simulink model "Project_4_Simulation"  (R2023b)
settings: Solver=VariableStepAuto  StartTime=0.0  StopTime=10.0  RelTol=1e-3
undefined symbols (not defined in the file or in its folder): batData, carData, motorData, track_radius
libraries: slpidlib x1
settings Model: Creator=mccal  LastModifiedBy=mccal

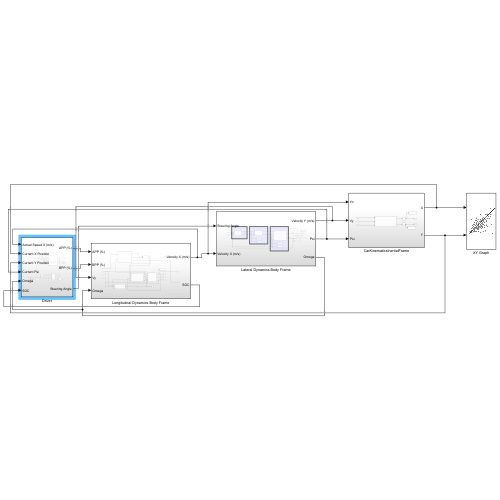
[thumbnail: Simulink's stored preview of the top-level diagram]
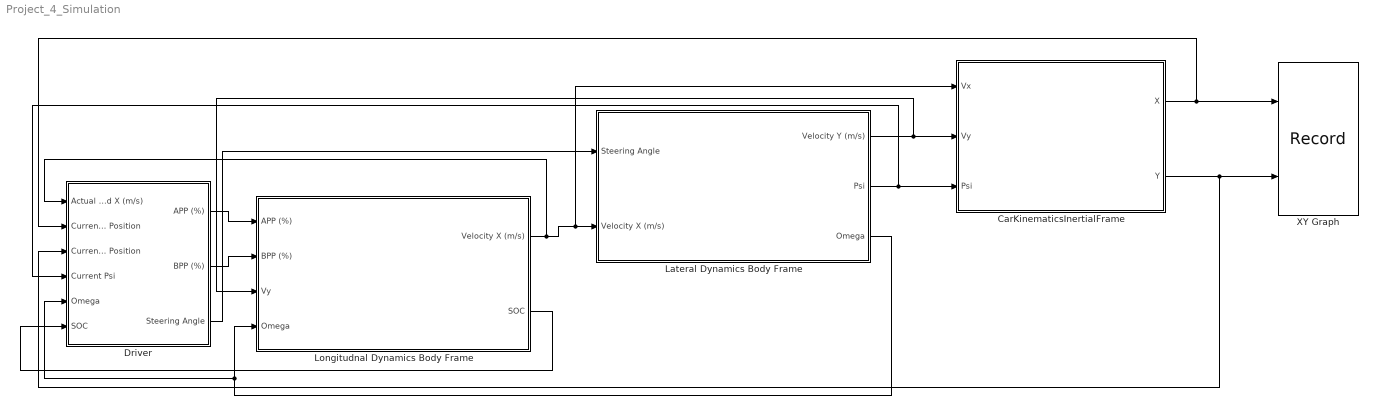
== system Project_4_Simulation ==
  CarKinematicsInertialFrame : Subsystem
  Driver : Subsystem
  Lateral Dynamics Body Frame : Subsystem
  Longitudnal Dynamics Body Frame : Subsystem
  XY Graph : Record  FileSettingsInternal="{\"entries\":[{\"content\":{\"excelSettings\":{\"content\":{},\"type\":\"Streamout.ExcelSettings\"}},\"type\":\"Streamout.FileSettingStorage\",\"uuid\":\"\"}],\"packageUris\":[\"http:\\/\\/schema.mathworks.com\\/mf0\\/streamout_blocks\\/R2020a\"],\"version\":\"1.0\"}"  Layout=[1 1]  SignalsInternal="{\"entries\":[{\"content\":{\"signals\":[{\"content\":{\"blockPath\":[],\"dimensions\":[1],\"domain\":\"\",\"lineColor\":\"#d95319\",\"port\":1,\"sid\":[\"\"],\"signalID\":3841,\"signalName\":\"CarKinematicsInertialFrame:1\"},\"type\":\"RecordBlkView.Signal\",\"uuid\":\"\"},{\"content\":{\"blockPath\":[],\"dimensions\":[1],\"domain\":\"\",\"lineColor\":\"#edb120\",\"port\":2,\"sid\":[\"\"],\"signalID\":3845,\"signalName\":\"CarKinematicsInertialFrame:2\"},\"type\":\"RecordBlkView.Signal\",\"uuid\":\"\"}]},\"type\":\"RecordBlkView.InputSignals\",\"uuid\":\"\"}],\"packageUris\":[\"http:\\/\\/schema.mathworks.com\\/mf0\\/streamout_blocks\\/R2020a\"],\"version\":\"1.0\"}"  VisualizationBindings="{\"xyplotplugin\":{\"info\":[{\"series\":[],\"subplotID\":1}]}}"  CompatibilityTag=XY  st=-1
  wires:
  CarKinematicsInertialFrame/2(Y) -> Driver/3(Current Y Position), XY Graph/2
  CarKinematicsInertialFrame/1(X) -> Driver/2(Current X Position), XY Graph/1
  Lateral Dynamics Body Frame/1(Velocity Y (m/s)) -> Longitudnal Dynamics Body Frame/3(Vy), CarKinematicsInertialFrame/2(Vy)
  Lateral Dynamics Body Frame/2(Psi) -> Driver/4(Current Psi), CarKinematicsInertialFrame/3(Psi)
  Driver/1(APP (%)) -> Longitudnal Dynamics Body Frame/1(APP (%))
  Driver/2(BPP (%)) -> Longitudnal Dynamics Body Frame/2(BPP (%))
  Longitudnal Dynamics Body Frame/1(Velocity X (m/s)) -> Driver/1(Actual Speed X (m/s)), CarKinematicsInertialFrame/1(Vx), Lateral Dynamics Body Frame/2(Velocity X (m/s))
  Lateral Dynamics Body Frame/3(Omega) -> Longitudnal Dynamics Body Frame/4(Omega), Driver/5(Omega)
  Longitudnal Dynamics Body Frame/2(SOC) -> Driver/6(SOC)
  Driver/3(Steering Angle) -> Lateral Dynamics Body Frame/1(Steering Angle)

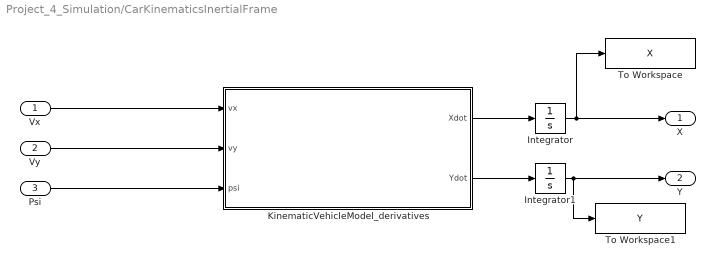
== system Project_4_Simulation/CarKinematicsInertialFrame ==
  Vx : Inport
  Vy : Inport  Port=2
  Psi : Inport  Port=3
  Integrator : Integrator  InitialCondition=carData.init.X0
  Integrator1 : Integrator  InitialCondition=carData.init.Y0
  KinematicVehicleModel_derivatives : MATLAB Function  TreatAsAtomicUnit=on  mask{obj=carData}
      mask prompts: obj "obj structure"
  To Workspace : ToWorkspace  VariableName=X  SaveFormat=Timeseries  SampleTime=-1
  To Workspace1 : ToWorkspace  VariableName=Y  SaveFormat=Timeseries  SampleTime=-1
  X : Outport
  Y : Outport  Port=2
  wires:
  KinematicVehicleModel_derivatives/1(Xdot) -> Integrator/1
  KinematicVehicleModel_derivatives/2(Ydot) -> Integrator1/1
  Integrator/1 -> To Workspace/1, X/1
  Integrator1/1 -> To Workspace1/1, Y/1
  Vx/1 -> KinematicVehicleModel_derivatives/1(vx)
  Vy/1 -> KinematicVehicleModel_derivatives/2(vy)
  Psi/1 -> KinematicVehicleModel_derivatives/3(psi)

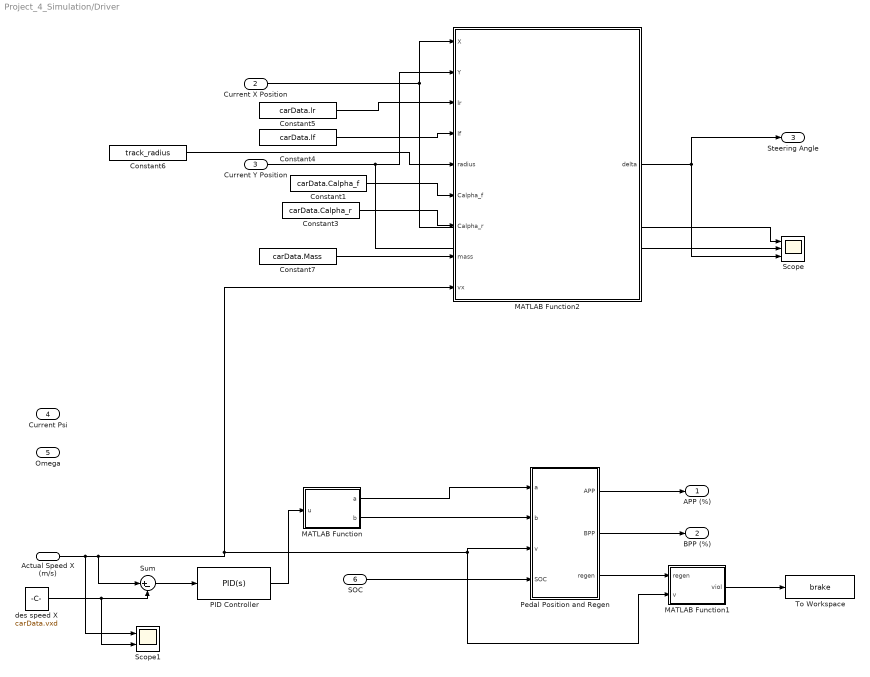
== system Project_4_Simulation/Driver ==
  Actual Speed X (m/s) : Inport
  Current X Position : Inport  Port=2
  Current Y Position : Inport  Port=3
  Current Psi : Inport  Port=4
  Omega : Inport  Port=5
  SOC : Inport  Port=6
  Constant1 : Constant  Value=carData.Calpha_f
  Constant3 : Constant  Value=carData.Calpha_r
  Constant4 : Constant  Value=carData.lf
  Constant5 : Constant  Value=carData.lr
  Constant6 : Constant  Value=track_radius
  Constant7 : Constant  Value=carData.Mass
  MATLAB Function : MATLAB Function  TreatAsAtomicUnit=on
  MATLAB Function1 : MATLAB Function  TreatAsAtomicUnit=on
  MATLAB Function2 : MATLAB Function  TreatAsAtomicUnit=on
  PID Controller : slpidlib/PID Controller  Controller=PID  Form=Parallel  TimeDomain=Continuous-time  UseExternalTs=off  SampleTime=-1  IntegratorMethod=Forward Euler  FilterMethod=Forward Euler  ControllerParametersSource=internal  P=1  I=0  UseKiTs=off  D=0  N=100  UseFilter=on  TunerSelectOption=Transfer Function Based (PID Tuner App)  InitialConditionSource=internal  InitialConditionForIntegrator=0  InitialConditionForFilter=0  DifferentiatorICPrevScaledInput=0  ExternalReset=none  TrackingMode=off  Kt=1  LimitOutput=on  SatLimitsSource=internal  UpperSaturationLimit=1  LowerSaturationLimit=-1  LinearizeAsGain=off  AntiWindupMode=none  Kb=1  LimitIntegrator=off  UpperIntegratorSaturationLimit=inf  LowerIntegratorSaturationLimit=-inf  POutMin=[]  POutMax=[]  IOutMin=[]  IOutMax=[]  DOutMin=[]  DOutMax=[]  NOutMin=[]  NOutMax=[]  SumOutMin=[]  SumOutMax=[]  SaturationOutMin=[]  SaturationOutMax=[]  PParamMin=[]  PParamMax=[]  IParamMin=[]  IParamMax=[]  DParamMin=[]  DParamMax=[]  NParamMin=[]  NParamMax=[]  KbParamMin=[]  KbParamMax=[]  KtParamMin=[]  KtParamMax=[]  KbOutMin=[]  KbOutMax=[]  KtOutMin=[]  KtOutMax=[]  IntegratorOutMin=[]  IntegratorOutMax=[]  FilterOutMin=[]  FilterOutMax=[]  SumI1OutMin=[]  SumI1OutMax=[]  SumI2OutMin=[]  SumI2OutMax=[]  SumI3OutMin=[]  SumI3OutMax=[]  SumI4OutMin=[]  SumI4OutMax=[]  SumDOutMin=[]  SumDOutMax=[]  DifferentiatorOutMin=[]  DifferentiatorOutMax=[]  FilterDiffOutCoefMin=[]  FilterDiffOutCoefMax=[]  ReciprocalOutMin=[]  ReciprocalOutMax=[]  SumDenOutMin=[]  SumDenOutMax=[]  SumNumOutMin=[]  SumNumOutMax=[]  DivideOutMin=[]  DivideOutMax=[]  UdiffTsProdOutMin=[]  UdiffTsProdOutMax=[]  NTsProdOutMin=[]  NTsProdOutMax=[]  UintegralTsProdOutMin=[]  UintegralTsProdOutMax=[]  UngainTsProdOutMin=[]  UngainTsProdOutMax=[]  ClampingZeroOutDataTypeStr=Inherit: Inherit via back propagation  ClampingZeroOutMin=[]  ClampingZeroOutMax=[]  FilterDenConstantOutDataTypeStr=Inherit: Inherit via back propagation  FilterDenConstantOutMin=[]  FilterDenConstantOutMax=[]  PCopyOutDataTypeStr=Inherit: Inherit via back propagation  PCopyOutMin=[]  PCopyOutMax=[]  NCopyOutDataTypeStr=Inherit: Inherit via back propagation  NCopyOutMin=[]  NCopyOutMax=[]  IntegratorContinuousStateAttributes=''  IntegratorStateMustResolveToSignalObject=off  IntegratorRTWStateStorageClass=Auto  FilterContinuousStateAttributes=''  FilterStateMustResolveToSignalObject=off  FilterRTWStateStorageClass=Auto  ParallelPVariant=InternalParameters  IdealPVariant=Disabled  IVariant=InternalParameters  DVariant=InternalParameters  IntegratorVariant=Continuous  SatVariant=Enabled  AWVariant=Passthrough  PCopyVariant=Disabled  TRVariant=Disabled  FdbkBlocksVariant=Forward  IdealPFdbkVariant=Disabled  SatFdbkVariant=Disabled  DerivativeFilterVariant=ContFilter  NVariant=InternalParameters  NCopyVariant=Disabled  FilterICVariant=InternalICsFilter  IntegratorICVariant=InternalICs  ExternalResetVariant=Disabled  TRSumVariant=Passthrough  SumFdbkVariant=Disabled  SumVariant=Sum_PID  TsampFilterVariant=InternalTs  TsampNgainVariant=Passthrough  TsampIntegralVariant=Disabled_SignalSpec  ExternalSaturationOutDataTypeStr=Inherit: Same as second input
  Pedal Position and Regen : MATLAB Function  TreatAsAtomicUnit=on
  Scope : Scope  NumInputPorts=3
  Scope1 : Scope  NumInputPorts=2
  Sum : Sum  Inputs=|+-
  To Workspace : ToWorkspace  VariableName=brake  SaveFormat=Timeseries  SampleTime=-1
  des speed X : Constant  Value=carData.vxd
  APP (%) : Outport
  BPP (%) : Outport  Port=2
  Steering Angle : Outport  Port=3
  wires:
  Pedal Position and Regen/1(APP) -> APP (%)/1
  Pedal Position and Regen/2(BPP) -> BPP (%)/1
  Pedal Position and Regen/3(regen) -> MATLAB Function1/1(regen)
  MATLAB Function1/1(viol) -> To Workspace/1
  Current X Position/1 -> Scope/1, MATLAB Function2/1(X)
  Constant3/1 -> MATLAB Function2/7(Calpha_r)
  Current Y Position/1 -> Scope/2, MATLAB Function2/2(Y)
  Constant1/1 -> MATLAB Function2/6(Calpha_f)
  Constant6/1 -> MATLAB Function2/5(radius)
  Constant5/1 -> MATLAB Function2/3(lr)
  Constant7/1 -> MATLAB Function2/8(mass)
  MATLAB Function2/1(delta) -> Steering Angle/1, Scope/3
  Constant4/1 -> MATLAB Function2/4(lf)
  SOC/1 -> Pedal Position and Regen/4(SOC)
  Actual Speed X (m/s)/1 -> Scope1/1, Sum/1, MATLAB Function2/9(vx), Pedal Position and Regen/3(v), MATLAB Function1/2(v)
  MATLAB Function/1(a) -> Pedal Position and Regen/1(a)
  MATLAB Function/2(b) -> Pedal Position and Regen/2(b)
  Sum/1 -> PID Controller/1
  des speed X/1 -> Scope1/2, Sum/2
  PID Controller/1 -> MATLAB Function/1(u)

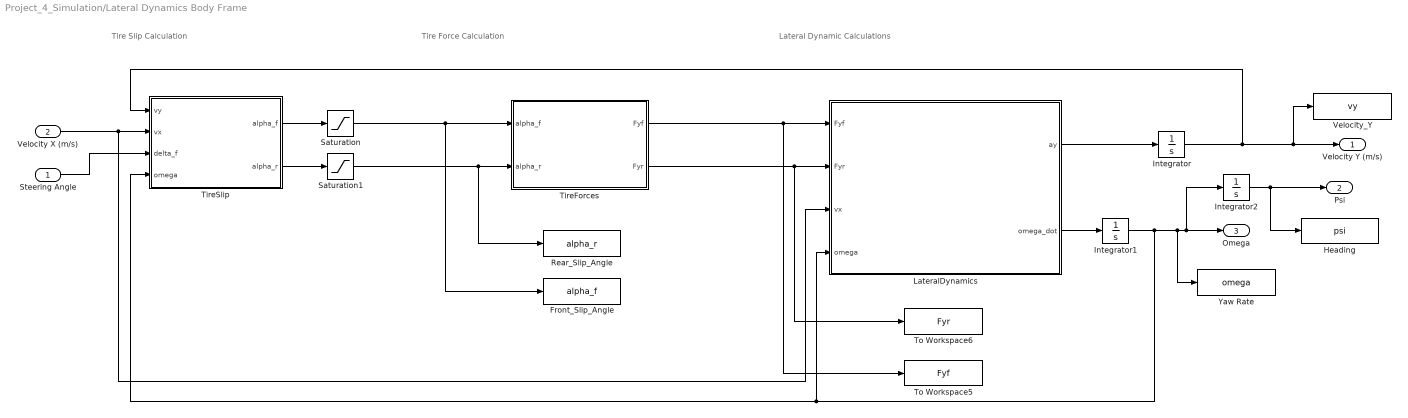
== system Project_4_Simulation/Lateral Dynamics Body Frame ==
  note: Tire Slip Calculation
  note: Tire Force Calculation
  note: Lateral Dynamic Calculations
  Steering Angle : Inport
  Velocity X (m/s) : Inport  Port=2
  Front_Slip_Angle : ToWorkspace  VariableName=alpha_f  SaveFormat=Timeseries  SampleTime=-1
  Heading : ToWorkspace  VariableName=psi  SaveFormat=Timeseries  SampleTime=-1
  Integrator : Integrator  InitialCondition=carData.init.vy0
  Integrator1 : Integrator  InitialCondition=carData.init.omega0
  Integrator2 : Integrator  InitialCondition=carData.init.psi0
  LateralDynamics : MATLAB Function  TreatAsAtomicUnit=on  mask{obj=carData}
      mask prompts: obj "obj structure"
  Rear_Slip_Angle : ToWorkspace  VariableName=alpha_r  SaveFormat=Timeseries  SampleTime=-1
  Saturation : Saturate  UpperLimit=carData.maxAlpha  LowerLimit=-carData.maxAlpha
  Saturation1 : Saturate  UpperLimit=carData.maxAlpha  LowerLimit=-carData.maxAlpha
  TireForces : MATLAB Function  TreatAsAtomicUnit=on  mask{obj=carData}
      mask prompts: obj "obj structure"
  TireSlip : MATLAB Function  TreatAsAtomicUnit=on  mask{obj=carData}
      mask prompts: obj "obj structure"
  To Workspace5 : ToWorkspace  VariableName=Fyf  SaveFormat=Timeseries  SampleTime=-1
  To Workspace6 : ToWorkspace  VariableName=Fyr  SaveFormat=Timeseries  SampleTime=-1
  Velocity_Y : ToWorkspace  VariableName=vy  SaveFormat=Timeseries  SampleTime=-1
  Yaw Rate : ToWorkspace  VariableName=omega  SaveFormat=Timeseries  SampleTime=-1
  Velocity Y (m/s) : Outport
  Psi : Outport  Port=2
  Omega : Outport  Port=3
  wires:
  LateralDynamics/1(ay) -> Integrator/1
  Integrator/1 -> Velocity Y (m/s)/1, Velocity_Y/1, TireSlip/1(vy)
  LateralDynamics/2(omega_dot) -> Integrator1/1
  Integrator1/1 -> Integrator2/1, Omega/1, Yaw Rate/1, LateralDynamics/4(omega), TireSlip/4(omega)
  TireSlip/1(alpha_f) -> Saturation/1
  TireSlip/2(alpha_r) -> Saturation1/1
  TireForces/1(Fyf) -> LateralDynamics/1(Fyf), To Workspace5/1
  TireForces/2(Fyr) -> LateralDynamics/2(Fyr), To Workspace6/1
  Saturation/1 -> TireForces/1(alpha_f), Front_Slip_Angle/1
  Saturation1/1 -> TireForces/2(alpha_r), Rear_Slip_Angle/1
  Velocity X (m/s)/1 -> TireSlip/2(vx), LateralDynamics/3(vx)
  Steering Angle/1 -> TireSlip/3(delta_f)
  Integrator2/1 -> Heading/1, Psi/1

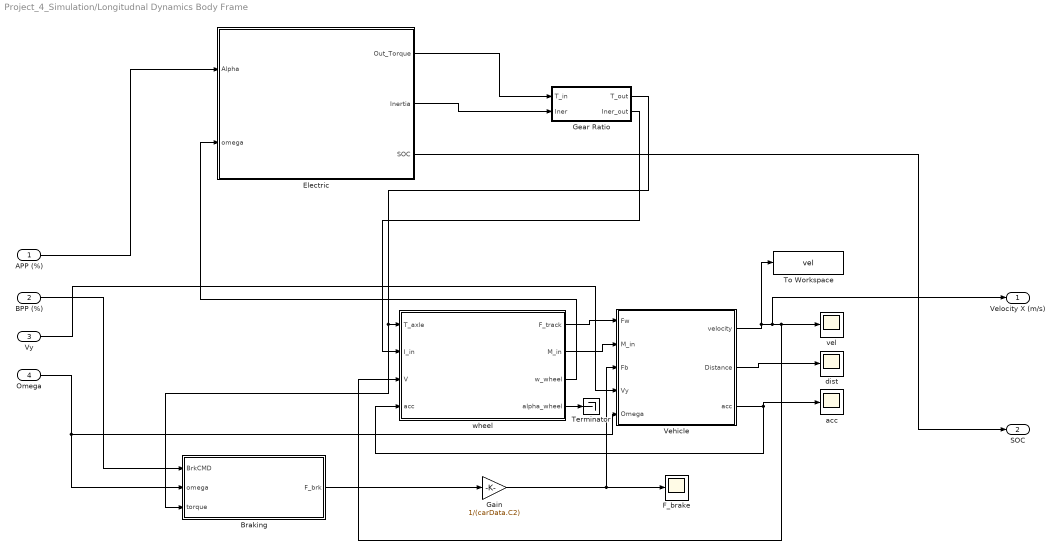
== system Project_4_Simulation/Longitudnal Dynamics Body Frame ==
  APP (%) : Inport
  BPP (%) : Inport  Port=2
  Vy : Inport  Port=3
  Omega : Inport  Port=4
  Braking : Subsystem
  Electric : Subsystem
  F_brake : Scope
  Gain : Gain  Gain=1/(carData.C2)
  Gear Ratio : Subsystem
  Terminator : Terminator
  To Workspace : ToWorkspace  VariableName=vel  SaveFormat=Timeseries  SampleTime=-1
  Vehicle : Subsystem
  acc : Scope
  dist : Scope
  vel : Scope
  "wheel " : Subsystem
  Velocity X (m/s) : Outport
  SOC : Outport  Port=2
  wires:
  "wheel "/1(F_track) -> Vehicle/1("Fw ")
  "wheel "/4(alpha_wheel) -> Terminator/1
  "wheel "/2(M_in) -> Vehicle/2("M_in ")
  Electric/1(Out_Torque) -> Gear Ratio/1(T_in)
  Vehicle/2("Distance ") -> dist/1
  Gear Ratio/1(T_out) -> Braking/3(torque), "wheel "/1(T_axle)
  Braking/1("F_brk ") -> Gain/1
  Electric/2(Inertia) -> Gear Ratio/2(Iner)
  Gear Ratio/2(Iner_out) -> "wheel "/2(I_in)
  Gain/1 -> Vehicle/3("Fb "), F_brake/1
  "wheel "/3(w_wheel) -> Electric/2(omega)
  Vehicle/1("velocity ") -> To Workspace/1, Velocity X (m/s)/1, vel/1, "wheel "/3(V)
  Vehicle/3(acc) -> acc/1, "wheel "/4(acc)
  BPP (%)/1 -> Braking/1("BrkCMD ")
  APP (%)/1 -> Electric/1(Alpha)
  Omega/1 -> Vehicle/5(Omega), Braking/2("omega ")
  Vy/1 -> Vehicle/4(Vy)
  Electric/3(SOC) -> SOC/1

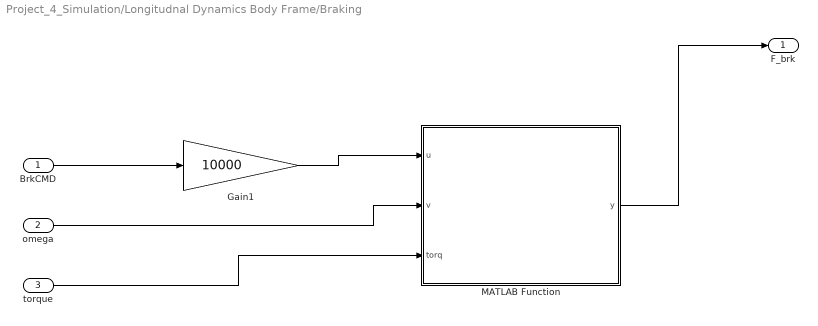
== system Project_4_Simulation/Longitudnal Dynamics Body Frame/Braking ==
  "BrkCMD " : Inport
  "omega " : Inport  Port=2
  torque : Inport  Port=3
  Gain1 : Gain  Gain=10000
  MATLAB Function : MATLAB Function  TreatAsAtomicUnit=on
  "F_brk " : Outport  VectorParamsAs1DForOutWhenUnconnected=off
  wires:
  "BrkCMD "/1 -> Gain1/1
  Gain1/1 -> MATLAB Function/1(u)
  MATLAB Function/1(y) -> "F_brk "/1
  "omega "/1 -> MATLAB Function/2(v)
  torque/1 -> MATLAB Function/3(torq)

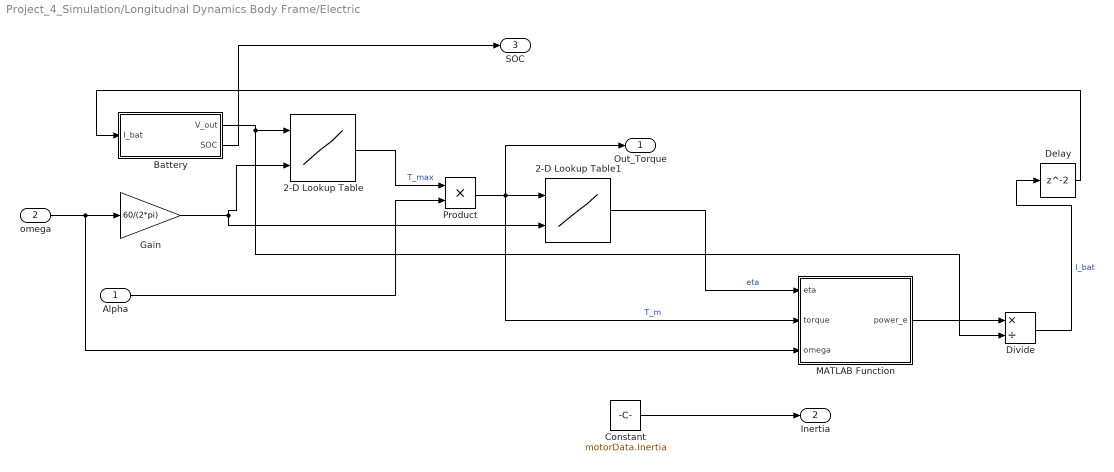
== system Project_4_Simulation/Longitudnal Dynamics Body Frame/Electric ==
  Alpha : Inport
  omega : Inport  Port=2
  2-D Lookup Table : Lookup_n-D  BreakpointsForDimension1=motorData.vbus  BreakpointsForDimension2=motorData.rpm  Table=motorData.maxtorque  InternalRulePriority=Speed  RndMeth=Simplest
      settings: InputPortMap=u0,u1
  2-D Lookup Table1 : Lookup_n-D  BreakpointsForDimension1=motorData.eta_torque  BreakpointsForDimension2=motorData.eta_speed  Table=motorData.eta_val  InternalRulePriority=Speed  RndMeth=Simplest
      settings: InputPortMap=u0,u1
  Battery : Subsystem
  Constant : Constant  Value=motorData.Inertia
  Delay : Delay
  Divide : Product  Inputs=*/
  Gain : Gain  Gain=60/(2*pi)
  MATLAB Function : MATLAB Function  TreatAsAtomicUnit=on
  Product : Product
  Out_Torque : Outport
  Inertia : Outport  Port=2
  SOC : Outport  Port=3
  wires:
  2-D Lookup Table/1 -> Product/1  "T_max"
  Alpha/1 -> Product/2
  Product/1 -> Out_Torque/1, MATLAB Function/2(torque), 2-D Lookup Table1/1  "T_m"
  Battery/1(V_out) -> Divide/2, 2-D Lookup Table/1
  2-D Lookup Table1/1 -> MATLAB Function/1(eta)  "eta"
  omega/1 -> MATLAB Function/3(omega), Gain/1
  MATLAB Function/1(power_e) -> Divide/1
  Delay/1 -> Battery/1(I_bat)
  Gain/1 -> 2-D Lookup Table/2, 2-D Lookup Table1/2
  Constant/1 -> Inertia/1
  Battery/2(SOC) -> SOC/1
  Divide/1 -> Delay/1  "I_bat"

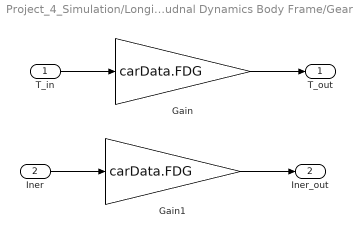
== system Project_4_Simulation/Longitudnal Dynamics Body Frame/Gear Ratio ==
  T_in : Inport
  Iner : Inport  Port=2
  Gain : Gain  Gain=carData.FDG
  Gain1 : Gain  Gain=carData.FDG
  T_out : Outport
  Iner_out : Outport  Port=2
  wires:
  T_in/1 -> Gain/1
  Gain/1 -> T_out/1
  Iner/1 -> Gain1/1
  Gain1/1 -> Iner_out/1

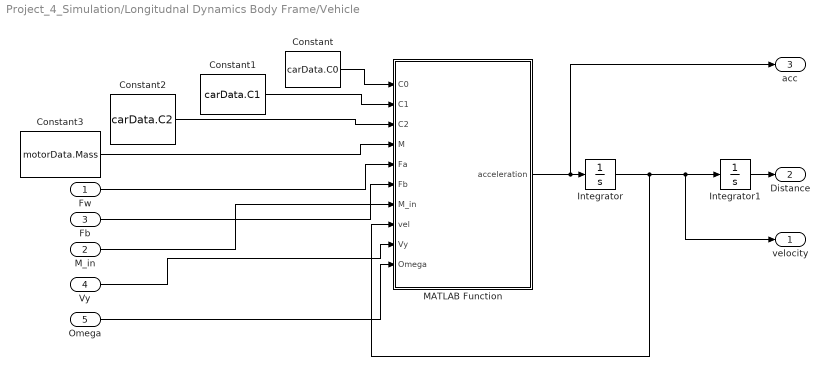
== system Project_4_Simulation/Longitudnal Dynamics Body Frame/Vehicle ==
  "Fw " : Inport
  "M_in " : Inport  Port=2
  "Fb " : Inport  Port=3
  Vy : Inport  Port=4
  Omega : Inport  Port=5
  Constant : Constant  Value=carData.C0
  Constant1 : Constant  Value=carData.C1
  Constant2 : Constant  Value=carData.C2
  Constant3 : Constant  Value=motorData.Mass
  Integrator : Integrator  LimitOutput=on  LowerSaturationLimit=0
  Integrator1 : Integrator
  MATLAB Function : MATLAB Function  TreatAsAtomicUnit=on
  "velocity " : Outport  VectorParamsAs1DForOutWhenUnconnected=off
  "Distance " : Outport  Port=2  VectorParamsAs1DForOutWhenUnconnected=off
  acc : Outport  Port=3
  wires:
  Constant1/1 -> MATLAB Function/2(C1)
  Constant/1 -> MATLAB Function/1(C0)
  MATLAB Function/1(acceleration) -> acc/1, Integrator/1
  Constant2/1 -> MATLAB Function/3(C2)
  Constant3/1 -> MATLAB Function/4(M)
  "Fw "/1 -> MATLAB Function/5(Fa)
  "Fb "/1 -> MATLAB Function/6(Fb)
  Integrator/1 -> MATLAB Function/8(vel), "velocity "/1, Integrator1/1
  Integrator1/1 -> "Distance "/1
  "M_in "/1 -> MATLAB Function/7(M_in)
  Vy/1 -> MATLAB Function/9(Vy)
  Omega/1 -> MATLAB Function/10(Omega)

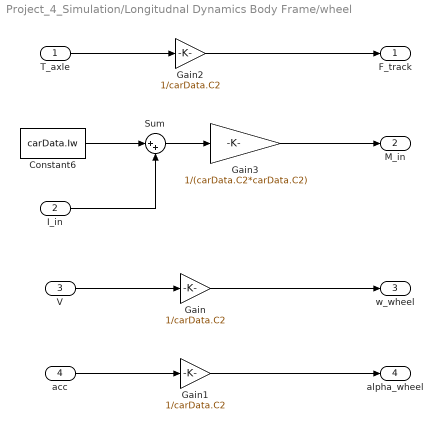
== system Project_4_Simulation/Longitudnal Dynamics Body Frame/wheel  ==
  T_axle : Inport
  I_in : Inport  Port=2
  V : Inport  Port=3
  acc : Inport  Port=4
  Constant6 : Constant  Value=carData.Iw
  Gain : Gain  Gain=1/carData.C2
  Gain1 : Gain  Gain=1/carData.C2
  Gain2 : Gain  Gain=1/carData.C2
  Gain3 : Gain  Gain=1/(carData.C2*carData.C2)
  Sum : Sum  Inputs=|++
  F_track : Outport
  M_in : Outport  Port=2
  w_wheel : Outport  Port=3
  alpha_wheel : Outport  Port=4
  wires:
  Gain/1 -> w_wheel/1
  V/1 -> Gain/1
  acc/1 -> Gain1/1
  Gain1/1 -> alpha_wheel/1
  T_axle/1 -> Gain2/1
  Gain2/1 -> F_track/1
  Gain3/1 -> M_in/1
  Constant6/1 -> Sum/1
  I_in/1 -> Sum/2
  Sum/1 -> Gain3/1

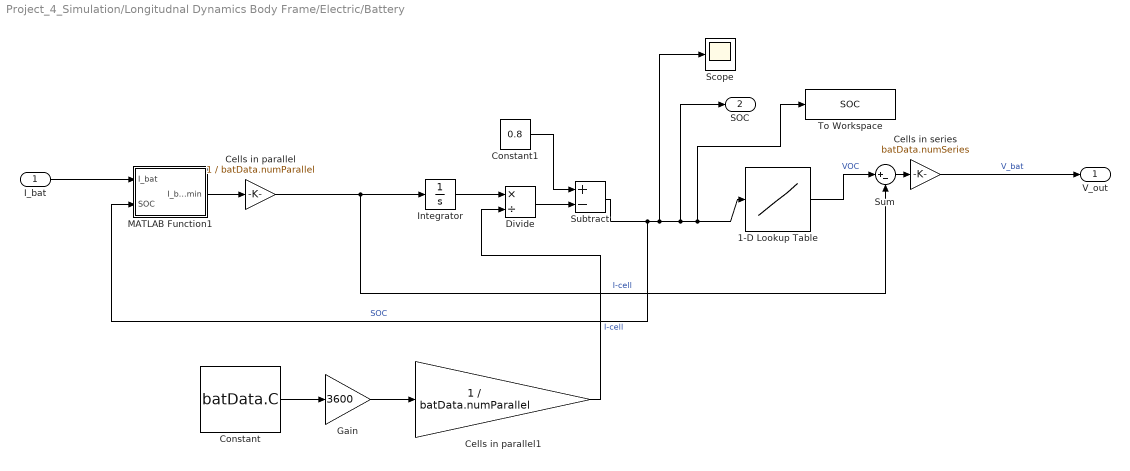
== system Project_4_Simulation/Longitudnal Dynamics Body Frame/Electric/Battery ==
  I_bat : Inport
  1-D Lookup Table : Lookup_n-D  NumberOfTableDimensions=1  BreakpointsForDimension1=batData.SOC  Table=batData.OCV  InternalRulePriority=Speed  RndMeth=Simplest
  Cells in parallel : Gain  Gain=1 / batData.numParallel
  Cells in parallel1 : Gain  Gain=1 / batData.numParallel
  Cells in series : Gain  Gain=batData.numSeries
  Constant : Constant  Value=batData.C
  Constant1 : Constant  Value=0.8
  Divide : Product  Inputs=*/
  Gain : Gain  Gain=3600
  Integrator : Integrator
  MATLAB Function1 : MATLAB Function  TreatAsAtomicUnit=on
  Scope : Scope
  Subtract : Sum  Inputs=+-
  Sum : Sum  Inputs=|+-
  To Workspace : ToWorkspace  VariableName=SOC  SaveFormat=Timeseries  SampleTime=-1
  V_out : Outport
  SOC : Outport  Port=2
  wires:
  1-D Lookup Table/1 -> Sum/1  "VOC"
  Cells in series/1 -> V_out/1  "V_bat"
  Sum/1 -> Cells in series/1
  Cells in parallel/1 -> Integrator/1, Sum/2  "I-cell"
  Integrator/1 -> Divide/1
  Constant/1 -> Gain/1
  Constant1/1 -> Subtract/1
  Divide/1 -> Subtract/2
  Subtract/1 -> 1-D Lookup Table/1, To Workspace/1, SOC/1, Scope/1, MATLAB Function1/2(SOC)  "SOC"
  Gain/1 -> Cells in parallel1/1
  Cells in parallel1/1 -> Divide/2  "I-cell"
  MATLAB Function1/1(I_bat_min) -> Cells in parallel/1
  I_bat/1 -> MATLAB Function1/1(I_bat)

== matlab function Project_4_Simulation/Driver/MATLAB Function1 ==
  data: regen input; viol output; v input
function viol = fcn(regen, v)

speed = (3600/1600)*v;
    if speed < 5
        regen_vio = 0;
        if regen == regen_vio
            viol = 0;
        else
            viol = 1;
        end

    elseif speed == 25
        regen_vio = 0.95;
        if regen == regen_vio
            viol = 0;
        else
            viol = 1;
        end

    elseif speed > 25
        regen_vio = 0.95;
        if regen == regen_vio
            viol = 0;
        else
            viol = 1;
        end
    else
        regen_vio = ((0.95/20)*speed) - 0.2375;
        if regen == regen_vio
            viol = 0;
        else
            viol = 1;
        end
    end

== matlab function Project_4_Simulation/Driver/MATLAB Function2 ==
  data: X input; delta output; Y input; lr input; lf input; radius input; Calpha_f input; Calpha_r input; mass input; vx input
function delta = SimplestDriver(X,Y, lr, lf, radius, Calpha_f, Calpha_r, mass, vx)

%===============================
total_length = lr + lf;
temp_front = lf / Calpha_f;
temp_rear = lr / Calpha_r;
temp_together = mass * vx * vx * (temp_rear - temp_front) / (total_length * radius);
kp = 0.001; 

if X > 900
    delta = (total_length) / (radius) + temp_together;
    error = sqrt((X - 900)^2 + (Y - 200)^2) - radius;
    delta = delta + kp * error;
elseif X < 0
    delta = (total_length) / (radius) + temp_together;
    error = sqrt((X)^2 + (Y - 200)^2) - radius;
    delta = delta + kp * error;
elseif Y < 200
    delta = 0;
    error = -Y;
    delta = delta + kp * error;
else
    delta = 0;
    error = Y - 400;
    delta = delta + kp * error;
end

== matlab function Project_4_Simulation/Driver/MATLAB Function ==
  data: u input; a output; b output
function [a,b] = fcn(u)

if u>0
    acc=u;
    brk=0;
elseif u<0
    acc=0;
    brk=u;
else
    acc=0;
    brk=0;
end
a= acc;
b= brk;

== matlab function Project_4_Simulation/Longitudnal Dynamics Body Frame/Electric/Battery/MATLAB Function1 ==
  data: I_bat input; I_bat_min output; SOC input
function I_bat_min = fcn(I_bat, SOC)

if (SOC >= 0.95) && (SOC<= 0.1)
    I_bat_min = 0;
else 
    I_bat_min = I_bat;
end

== matlab function Project_4_Simulation/Lateral Dynamics Body Frame/LateralDynamics ==
  data: Fyf input; Fyr input size=1; vx input; omega input; ay output; obj parameter; omega_dot output
function [ay, omega_dot] = fcn(Fyf, Fyr, vx, omega, obj)

Fy = Fyf + Fyr;
ay = Fy / obj.Mass - omega * vx;
        
M  = Fyf * obj.lf - Fyr * obj.lr;        
omega_dot = M / obj.Inertia;        

end

== matlab function Project_4_Simulation/Longitudnal Dynamics Body Frame/Braking/MATLAB Function ==
  data: u input; y output; v input; torq input
function y = fcn(u,v, torq)
if v == 0
    y = -min(abs(torq), u) *  torq/(abs(torq)+0.001);
else
    y = -(u * v/(abs(v)+0.001));
end

== matlab function Project_4_Simulation/CarKinematicsInertialFrame/KinematicVehicleModel_derivatives ==
  data: vx input; vy input; psi input size=1; Xdot output; Ydot output
function [Xdot, Ydot] = fcn(vx, vy, psi)
    temp = TF(psi) * [vx;vy]; 
    Xdot = temp(1);
    Ydot = temp(2);
  
end

function y = TF(psi)
    y = [cos(psi), -sin(psi); sin(psi), cos(psi)];
end

== matlab function Project_4_Simulation/Longitudnal Dynamics Body Frame/Vehicle/MATLAB Function ==
  data: C0 input; acceleration output; C1 input; C2 input; M input; Fa input; Fb input; M_in input; vel input; Vy input; Omega input
function acceleration   = vehicle(C0,C1,C2,M,Fa,Fb,M_in, vel, Vy, Omega)

acceleration = (((Fa-Fb))-(C0+ C1*vel + C2*(vel)^2))/(M+M_in) + (Vy*Omega);

== matlab function Project_4_Simulation/Longitudnal Dynamics Body Frame/Electric/MATLAB Function ==
  data: eta input; power_e output; torque input; omega input
function power_e = fcn(eta, torque, omega)
power_m = torque * omega;
sign_eta = power_m/(abs(power_m)+0.001);
power_e = power_m * eta^(sign_eta);

== matlab function Project_4_Simulation/Lateral Dynamics Body Frame/TireSlip ==
  data: vy input size=1; vx input; delta_f input size=1; omega input; alpha_f output; obj parameter; alpha_r output
function [alpha_f, alpha_r] = fcn(vy,  vx, delta_f, omega, obj)


if abs(vx)> obj.vx_threshold1
      alpha_f = delta_f - (vy + omega * obj.lf) / vx;
      alpha_r = - (vy - omega * obj.lr) / vx;
else
      alpha_f = 0;
      alpha_r = 0;
end



end

== matlab function Project_4_Simulation/Lateral Dynamics Body Frame/TireForces ==
  data: alpha_f input; alpha_r input; Fyf output; obj parameter; Fyr output
function [Fyf, Fyr] = fcn(alpha_f, alpha_r, obj)

Fyf = min(obj.Fyfmax,obj.Calpha_f * alpha_f);
Fyr = min(obj.Fyrmax, obj.Calpha_r * alpha_r);
end

== matlab function Project_4_Simulation/Driver/Pedal Position and Regen ==
  data: a input; APP output; b input; v input; SOC input; BPP output; regen output
function [APP, BPP, regen] = fcn(a, b, v, SOC)

APP = a + (b *.15);

BPP = b * .85;

speed = (3600/1600)*v;
if (speed <= 5)
    regen = 0;
elseif (speed > 5) && (speed < 25)
    regen =  ((0.95/20)*speed) - 0.2375;
else 
    regen = .95;
end
